simulink model "stateflow_1_stm"  (R2021b)
settings: Solver=VariableStepAuto  StartTime=0.0  StopTime=10.0  RelTol=1e-3
settings Model: Creator=fredric  LastModifiedBy=fredric

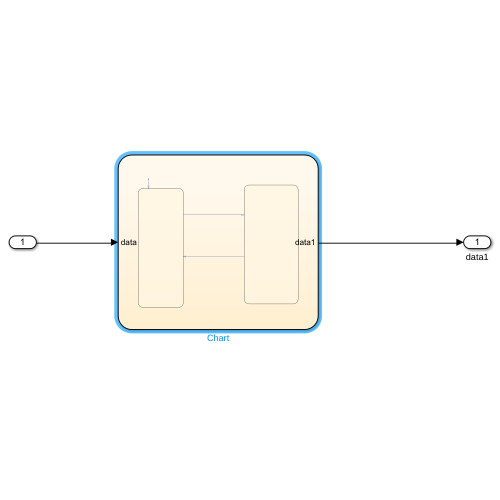
[thumbnail: Simulink's stored preview of the top-level diagram]
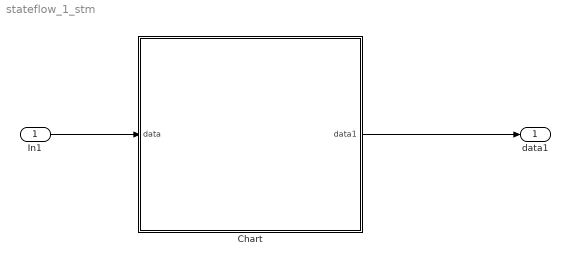
== system stateflow_1_stm ==
  In1 : Inport
  Chart : Stateflow chart  TreatAsAtomicUnit=on
  data1 : Outport
  wires:
  In1/1 -> Chart/1(data)
  Chart/1(data1) -> data1/1

== stateflow chart stateflow_1_stm/Chart ==
  state B
  state A
    en:
    output = 2;
    du:
    output = 2;
    ex:
    output = 0;
  (default) -> A
  A -> B : [input ==  1]
  B -> A : [input == 2]
  data: data input; data1 output
